simulink model "grafica1"  (R2021a)
settings: Solver=VariableStepAuto  StartTime=0.0  StopTime=10.0  RelTol=1e-3
settings Model: Creator=andrea  LastModifiedBy=andrea

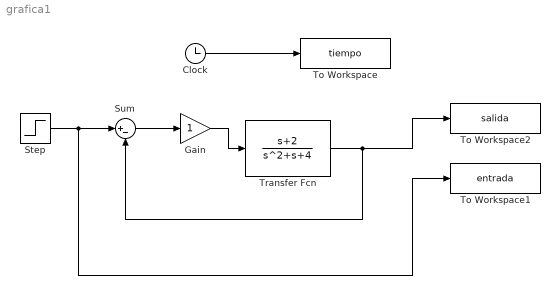
== system grafica1 ==
  Clock : Clock
  Gain : Gain
  Step : Step  SampleTime=0
  Sum : Sum  Inputs=|+-
  To Workspace : ToWorkspace  VariableName=tiempo  SampleTime=-1
  To Workspace1 : ToWorkspace  VariableName=entrada  SampleTime=-1
  To Workspace2 : ToWorkspace  VariableName=salida  SampleTime=-1
  Transfer Fcn : TransferFcn  Numerator=[1 2]  Denominator=[1 1 4]
  wires:
  Step/1 -> To Workspace1/1, Sum/1
  Transfer Fcn/1 -> To Workspace2/1, Sum/2
  Sum/1 -> Gain/1
  Gain/1 -> Transfer Fcn/1
  Clock/1 -> To Workspace/1
